simulink model "MbFu"  (R2018b)
settings: Solver=VariableStepAuto  StartTime=0.0  StopTime=1  RelTol=1e-3
settings Model: Creator=kekos  LastModifiedBy=kekos

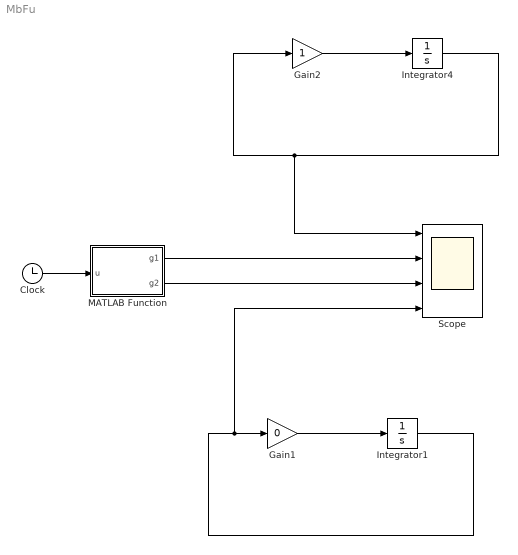
== system MbFu ==
  Clock : Clock
  Gain1 : Gain  Gain=0
  Gain2 : Gain
  Integrator1 : Integrator  InitialCondition=4*exp(-4)
  Integrator4 : Integrator  InitialCondition=3
  MATLAB Function : MATLAB Function  TreatAsAtomicUnit=on
  Scope : Scope  NumInputPorts=4
  wires:
  Clock/1 -> MATLAB Function/1(u)
  MATLAB Function/2(g2) -> Scope/3
  Gain2/1 -> Integrator4/1
  MATLAB Function/1(g1) -> Scope/2
  Integrator4/1 -> Scope/1, Gain2/1
  Gain1/1 -> Integrator1/1
  Integrator1/1 -> Scope/4, Gain1/1

== matlab function MbFu/MATLAB Function ==
  data: u input; g1 output; g2 output
function [g1,g2] = fcn(u)

g2 = 3*exp(u);
g1 = 4*exp(-4) + 0*u;
